simulink model "gimbal_kinematics_model_10122019"  (R2018b)
settings: Solver=VariableStepAuto  StartTime=0.0  StopTime=20  RelTol=1e-3
libraries: simulink x1
settings Model: Creator=Paweł Tymiński  LastModifiedBy=Paweł Tymiński

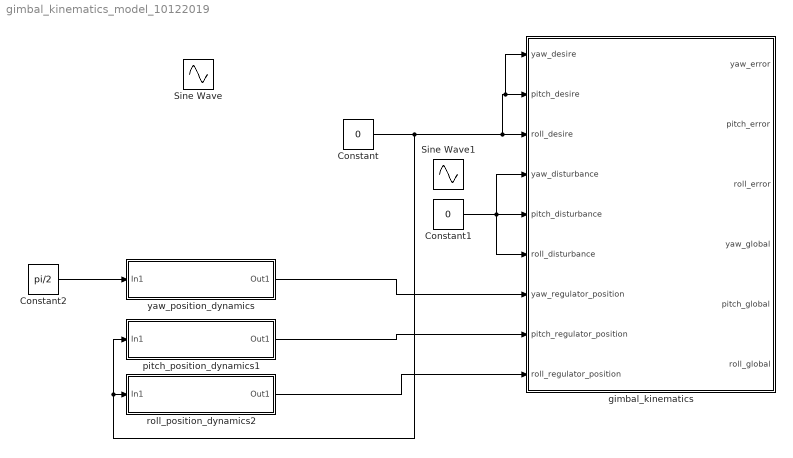
== system gimbal_kinematics_model_10122019 ==
  Constant : Constant  Value=0
  Constant1 : Constant  Value=0
  Constant2 : Constant  Value=pi/2
  Sine Wave : Sin  Amplitude=0.5  Frequency=0.5  SampleTime=0
  Sine Wave1 : Sin  Amplitude=0.5  Frequency=0.5  SampleTime=0
  gimbal_kinematics : Subsystem
  pitch_position_dynamics1 : Subsystem
  roll_position_dynamics2 : Subsystem
  yaw_position_dynamics : Subsystem
  wires:
  pitch_position_dynamics1/1(Out1) -> gimbal_kinematics/8(pitch_regulator_position)
  roll_position_dynamics2/1(Out1) -> gimbal_kinematics/9(roll_regulator_position)
  yaw_position_dynamics/1(Out1) -> gimbal_kinematics/7(yaw_regulator_position)
  Constant/1 -> roll_position_dynamics2/1(In1), pitch_position_dynamics1/1(In1), gimbal_kinematics/1(yaw_desire), gimbal_kinematics/2(pitch_desire), gimbal_kinematics/3(roll_desire)
  Constant1/1 -> gimbal_kinematics/4(yaw_disturbance), gimbal_kinematics/5(pitch_disturbance), gimbal_kinematics/6(roll_disturbance)
  Constant2/1 -> yaw_position_dynamics/1(In1)

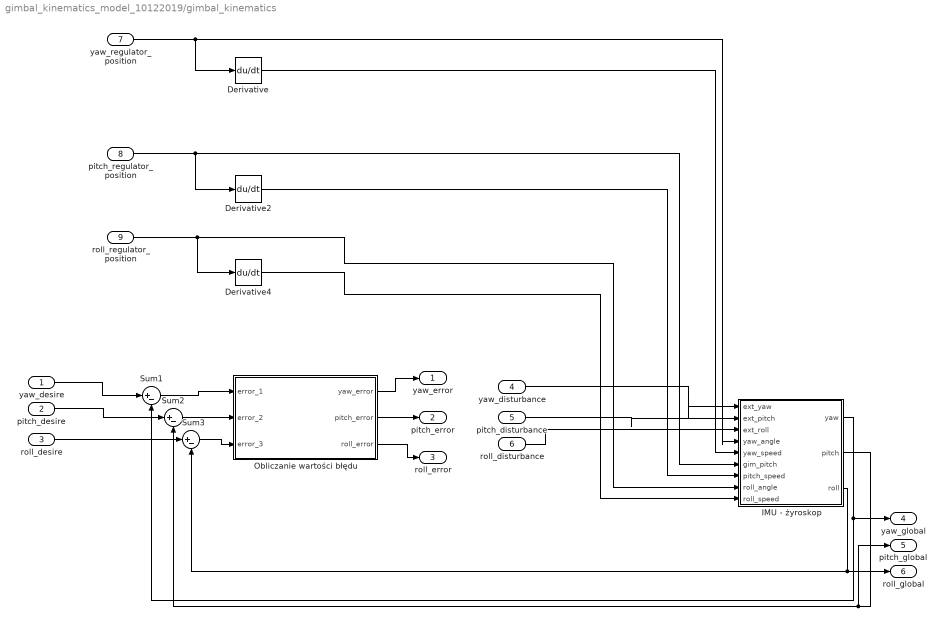
== system gimbal_kinematics_model_10122019/gimbal_kinematics ==
  yaw_desire : Inport
  pitch_desire : Inport  Port=2
  roll_desire : Inport  Port=3
  yaw_disturbance : Inport  Port=4
  pitch_disturbance : Inport  Port=5
  roll_disturbance : Inport  Port=6
  yaw_regulator_position : Inport  Port=7
  pitch_regulator_position : Inport  Port=8
  roll_regulator_position : Inport  Port=9
  Derivative : Derivative
  Derivative2 : Derivative
  Derivative4 : Derivative
  IMU - żyroskop : Subsystem
  Obliczanie wartości błędu : MATLAB Function  TreatAsAtomicUnit=on
  Sum1 : Sum  Inputs=|+-
  Sum2 : Sum  Inputs=|+-
  Sum3 : Sum  Inputs=|+-
  yaw_error : Outport
  pitch_error : Outport  Port=2
  roll_error : Outport  Port=3
  yaw_global : Outport  Port=4
  pitch_global : Outport  Port=5
  roll_global : Outport  Port=6
  wires:
  Sum3/1 -> Obliczanie wartości błędu/3(error_3)
  yaw_regulator_position/1 -> Derivative/1, IMU - żyroskop/4(yaw_angle)
  roll_regulator_position/1 -> Derivative4/1, IMU - żyroskop/8("roll_angle ")
  pitch_regulator_position/1 -> Derivative2/1, IMU - żyroskop/6(gim_pitch)
  IMU - żyroskop/2(pitch) -> Sum2/2, pitch_global/1
  Sum2/1 -> Obliczanie wartości błędu/2(error_2)
  Sum1/1 -> Obliczanie wartości błędu/1(error_1)
  pitch_disturbance/1 -> IMU - żyroskop/2(ext_pitch)
  IMU - żyroskop/3(roll) -> Sum3/2, roll_global/1
  IMU - żyroskop/1(yaw) -> Sum1/2, yaw_global/1
  Obliczanie wartości błędu/2(pitch_error) -> pitch_error/1
  roll_disturbance/1 -> IMU - żyroskop/3(ext_roll)
  yaw_disturbance/1 -> IMU - żyroskop/1(ext_yaw)
  Obliczanie wartości błędu/3(roll_error) -> roll_error/1
  Obliczanie wartości błędu/1(yaw_error) -> yaw_error/1
  yaw_desire/1 -> Sum1/1
  pitch_desire/1 -> Sum2/1
  roll_desire/1 -> Sum3/1
  Derivative/1 -> IMU - żyroskop/5(yaw_speed)
  Derivative2/1 -> IMU - żyroskop/7(pitch_speed)
  Derivative4/1 -> IMU - żyroskop/9(roll_speed)

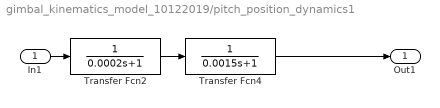
== system gimbal_kinematics_model_10122019/pitch_position_dynamics1 ==
  In1 : Inport
  Transfer Fcn2 : TransferFcn  Denominator=[0.0002 1]
  Transfer Fcn4 : TransferFcn  Denominator=[0.0015 1]
  Out1 : Outport
  wires:
  Transfer Fcn2/1 -> Transfer Fcn4/1
  In1/1 -> Transfer Fcn2/1
  Transfer Fcn4/1 -> Out1/1

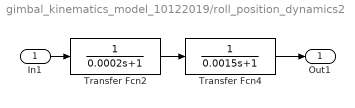
== system gimbal_kinematics_model_10122019/roll_position_dynamics2 ==
  In1 : Inport
  Transfer Fcn2 : TransferFcn  Denominator=[0.0002 1]
  Transfer Fcn4 : TransferFcn  Denominator=[0.0015 1]
  Out1 : Outport
  wires:
  Transfer Fcn2/1 -> Transfer Fcn4/1
  In1/1 -> Transfer Fcn2/1
  Transfer Fcn4/1 -> Out1/1

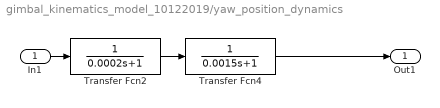
== system gimbal_kinematics_model_10122019/yaw_position_dynamics ==
  In1 : Inport
  Transfer Fcn2 : TransferFcn  Denominator=[0.0002 1]
  Transfer Fcn4 : TransferFcn  Denominator=[0.0015 1]
  Out1 : Outport
  wires:
  Transfer Fcn2/1 -> Transfer Fcn4/1
  In1/1 -> Transfer Fcn2/1
  Transfer Fcn4/1 -> Out1/1

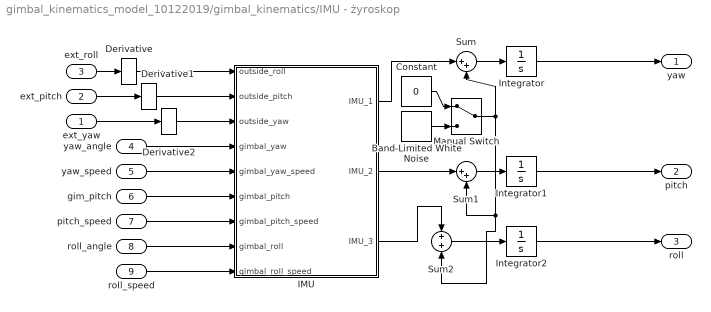
== system gimbal_kinematics_model_10122019/gimbal_kinematics/IMU - żyroskop ==
  ext_yaw : Inport
  ext_pitch : Inport  Port=2
  ext_roll : Inport  Port=3
  yaw_angle : Inport  Port=4
  yaw_speed : Inport  Port=5
  gim_pitch : Inport  Port=6
  pitch_speed : Inport  Port=7
  "roll_angle " : Inport  Port=8
  roll_speed : Inport  Port=9
  Band-Limited White Noise : simulink/Sources/Band-Limited White Noise  Cov=[0.1]  Ts=0.1  seed=[23341]
  Constant : Constant  Value=0
  Derivative : Derivative
  Derivative1 : Derivative
  Derivative2 : Derivative
  IMU : MATLAB Function  TreatAsAtomicUnit=on
  Integrator : Integrator
  Integrator1 : Integrator
  Integrator2 : Integrator
  Manual Switch : ManualSwitch
  Sum : Sum  Inputs=|++
  Sum1 : Sum  Inputs=|++
  Sum2 : Sum
  yaw : Outport
  pitch : Outport  Port=2
  roll : Outport  Port=3
  wires:
  roll_speed/1 -> IMU/9(gimbal_roll_speed)
  gim_pitch/1 -> IMU/6(gimbal_pitch)
  yaw_speed/1 -> IMU/5(gimbal_yaw_speed)
  IMU/1(IMU_1) -> Sum/1
  pitch_speed/1 -> IMU/7(gimbal_pitch_speed)
  ext_pitch/1 -> Derivative1/1
  ext_roll/1 -> Derivative/1
  ext_yaw/1 -> Derivative2/1
  "roll_angle "/1 -> IMU/8(gimbal_roll)
  yaw_angle/1 -> IMU/4(gimbal_yaw)
  IMU/3(IMU_3) -> Sum2/1
  IMU/2(IMU_2) -> Sum1/1
  Manual Switch/1 -> Sum2/2, Sum1/2, Sum/2
  Sum2/1 -> Integrator2/1
  Sum1/1 -> Integrator1/1
  Sum/1 -> Integrator/1
  Band-Limited White Noise/1 -> Manual Switch/2
  Constant/1 -> Manual Switch/1
  Derivative/1 -> IMU/1(outside_roll)
  Derivative1/1 -> IMU/2(outside_pitch)
  Derivative2/1 -> IMU/3(outside_yaw)
  Integrator/1 -> yaw/1
  Integrator2/1 -> roll/1
  Integrator1/1 -> pitch/1

== matlab function gimbal_kinematics_model_10122019/gimbal_kinematics/IMU - żyroskop/IMU ==
  data: outside_roll input; IMU_1 output; outside_pitch input; outside_yaw input; gimbal_yaw input; gimbal_yaw_speed input; gimbal_pitch input; gimbal_pitch_speed input; gimbal_roll input; gimbal_roll_speed input; IMU_2 output; IMU_3 output

function [IMU_1, IMU_2, IMU_3] = IMU(outside_roll,outside_pitch,outside_yaw,gimbal_yaw ,gimbal_yaw_speed, gimbal_pitch ,gimbal_pitch_speed , gimbal_roll , gimbal_roll_speed  )
% kąty gimbala
theta_1 = gimbal_yaw ;
theta_2 = gimbal_pitch ;
theta_3 = gimbal_roll ;

J_0 =[1 0 0;
    0 cos(theta_1) -sin(theta_1);
   -sin(theta_2) cos(theta_2)*sin(theta_1) cos(theta_1)*cos(theta_2)];
Phi_0 = [outside_yaw; outside_pitch; outside_roll];

Omega_phi = J_0*Phi_0;

Omega = [gimbal_yaw_speed; gimbal_pitch_speed; gimbal_roll_speed];

J = [cos(theta_2)*cos(theta_3) sin(theta_3) 0;
    cos(theta_2)*sin(theta_3) cos(theta_3) 0;
    -sin(theta_2) 0 1];
A=J*(Omega_phi + Omega);

IMU_1 = A(1); %yaw
IMU_2 = A(2); %pitch
IMU_3 = A(3); %roll

end

== matlab function gimbal_kinematics_model_10122019/gimbal_kinematics/Obliczanie wartości błędu ==
  data: error_1 input; error_2 input; error_3 input; yaw_error output; pitch_error output; roll_error output
function [yaw_error, pitch_error, roll_error] = fcn(error_1,error_2,error_3)
E=[cos(error_1)*cos(error_3)-sin(error_1)*sin(error_2)*sin(error_3) -cos(error_2)*sin(error_1) cos(error_1)*sin(error_1)+cos(error_3)*sin(error_1)*sin(error_2);
cos(error_3)*sin(error_1)+cos(error_1)*sin(error_2)*sin(error_2) cos(error_1)*cos(error_2) sin(error_1)*sin(error_3)-cos(error_1)*cos(error_3)*sin(error_2);
-cos(error_2)*sin(error_3) sin(error_2) cos(error_2)*cos(error_3)];



r12 = E(1,2);
r22 = E(2,2);
r31 = E(3,1);
r32 = E(3,2);
r33 = E(3,3);
yaw_D=atan2(-r12,r22);
pitch_D=asin(r32);
roll_D=atan2(-r31,r33);
% yaw_error=yaw_D-yaw_L;
% pitch_error=pitch_D-pitch_L;
% roll_error=roll_D-roll_L;

yaw_error=yaw_D;
pitch_error=pitch_D;
roll_error=roll_D;
end
